simulink model "Simple_pendulum_model"  (R2023b)
settings: Solver=VariableStepAuto  StartTime=0.0  StopTime=10  MaxStep=0.01  RelTol=1e-3
values from neighbouring files (symbols this model uses):
  b = m_p*l_p*r_a    (= 0.000461604)    [LQRJoe.m]    (also in LQRScript.m)
undefined symbols (not defined in the file or in its folder): J, L, m
settings Model: Creator=user  LastModifiedBy=Dell

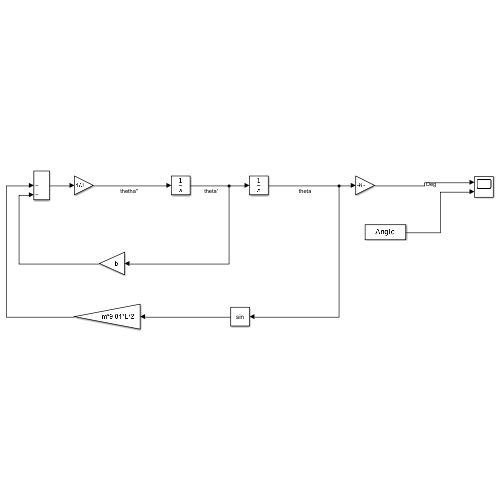
[thumbnail: Simulink's stored preview of the top-level diagram]
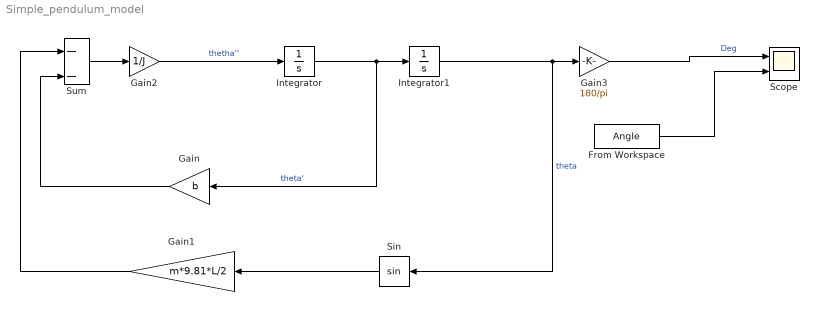
== system Simple_pendulum_model ==
  From Workspace : FromWorkspace  VariableName=Angle
  Gain : Gain  Gain=b
  Gain1 : Gain  Gain=m*9.81*L/2
  Gain2 : Gain  Gain=1/J
  Gain3 : Gain  Gain=180/pi
  Integrator : Integrator
  Integrator1 : Integrator  InitialCondition=1.6
  Scope : Scope  NumInputPorts=2
  Sin : Trigonometry
  Sum : Sum  Inputs=|--
  wires:
  Integrator/1 -> Gain/1, Integrator1/1  "theta'"
  Integrator1/1 -> Gain3/1, Sin/1  "theta"
  Gain2/1 -> Integrator/1  "thetha''"
  Gain1/1 -> Sum/1
  Sin/1 -> Gain1/1
  Gain/1 -> Sum/2
  Sum/1 -> Gain2/1
  Gain3/1 -> Scope/1  "Deg"
  From Workspace/1 -> Scope/2
